simulink model "uavPackageDelivery"  (R2025b)
settings: Solver=VariableStepAuto  StartTime=0.0  StopTime=simTime  FixedStep=.005  RelTol=1e-3  EnableMultiTasking=on
undefined symbols (not defined in the file): baseMission, Newton, oaMission, Raphson, uavIC_latLon, UAVSampleTime
libraries: robotcorelib x1, uavalgslib x1, visionsinks x1, robotalgslib x1
settings Model: DataDictionary=uavPackageDeliveryDataDict.sldd  ModifiedByFormat=The MathWorks, Inc.  PauseTimes=77  Creator=The MathWorks, Inc.  LastModifiedBy=The MathWorks, Inc.
settings SolverCC: AlgebraicLoopSolver=TrustRegion  AutoInsertRateTranBlk=on  MaxZcPerStep=1.0
settings DataIOCC: LimitDataPoints=on  ReturnWorkspaceOutputs=off
settings OptimizationCC: DefaultParameterBehavior=Inlined  DefaultUnderspecifiedDataType=single  EnhancedBackFolding=on  PassReuseOutputArgsThreshold=0.0  MaxStackSize=64  OptimizeBlockOrder=speed  DifferentSizesBufferReuse=on  OptimizationCustomize=off
settings DebuggingCC: ParameterPrecisionLossMsg=none  ParameterTunabilityLossMsg=error  UnconnectedInputMsg=warning  UnconnectedOutputMsg=warning  UnconnectedLineMsg=warning  AllowSymbolicDim=off  SFUnexpectedBacktrackingDiag=warning  SFNoUnconditionalDefaultTransitionDiag=warning  SFExecutionAtInitializationDiag=none  ArithmeticOperatorsInVariantConditions=warning
settings HardwareCC: ProdBitPerPointer=32.0  ProdBitPerSizeT=32.0  ProdBitPerPtrDiffT=32.0  ProdLargestAtomicFloat=None  ProdIntDivRoundTo=Undefined  ProdEndianess=Unspecified  ProdWordSize=32.0  ProdHWDeviceType=Generic->Unspecified (assume 32-bit Generic)
settings ModelReferenceCC: EnableRefExpFcnMdlSchedulingChecks=on  PropagateSignalLabelsOutOfModel=off
settings SFSimCC: SimUseLocalCustomCode=off  SimParseCustomCode=off  CustomCodeUndefinedFunction=UseInterfaceOnly
settings RTWCC: GenerateReport=on  RTWUseLocalCustomCode=off  LaunchReport=on  GPUComputeCapability=3.5  DLArmComputeVersion=19.05
settings CodeAppCC: ForceParamTrailComments=on  OperatorAnnotations=on
settings GRTTargetCC: TargetLangStandard=C89/C90 (ANSI)
settings ConfigComp: CovMetricSettings=dw  CovSaveCumulativeToWorkspaceVar=on  CovSaveSingleToWorkspaceVar=on  CovExternalEMLEnable=off

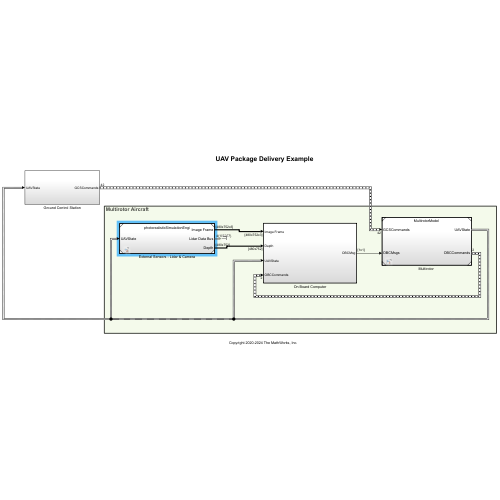
[thumbnail: Simulink's stored preview of the top-level diagram]
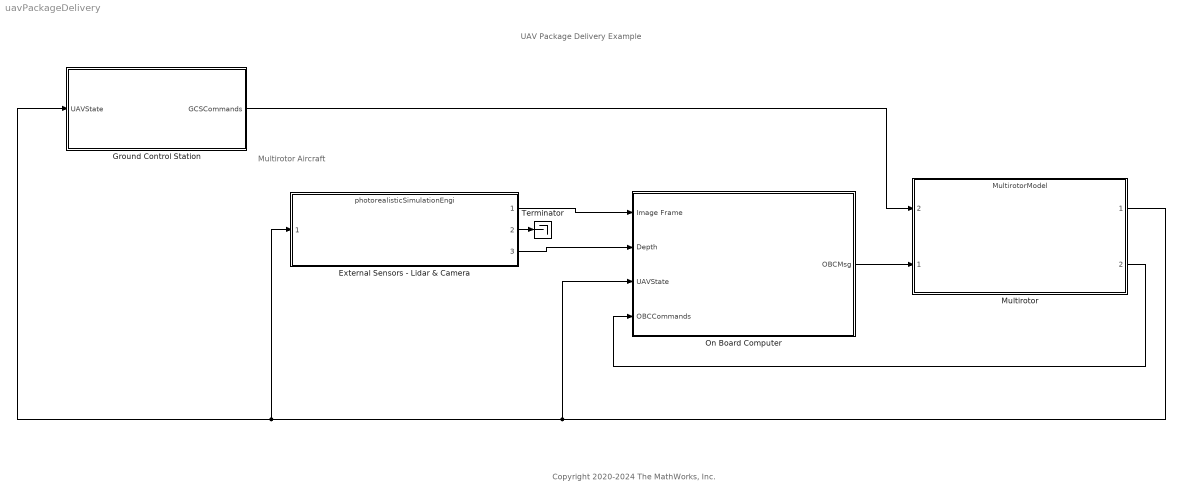
== system uavPackageDelivery ==
  note: Multirotor Aircraft
  note: UAV Package Delivery Example
  note: Copyright 2020-2024 The MathWorks, Inc.
  External Sensors - Lidar & Camera : ModelReference  ModelNameDialog=photorealisticSimulationEngi.slx  SimulationMode=Normal  ModelReferenceVersion=11.7
  Ground Control Station : Subsystem
  "Multirotor " : ModelReference  ModelNameDialog=MultirotorModel  SimulationMode=Normal  ModelReferenceVersion=12.1
      settings: PortSchema="{\"entries\":[{\"content\":{\"sides\":[{\"content\":{\"connectorIds\":[\"In2\",\"In1\"]},\"type\":\"ConnectorPlacement.EquallySpacedRectSide\",\"uuid\":\"abf53b88-b4c0-4cc3-bb4c-819ba68ade90\"},{\"content\":{\"connectorIds\":[\"Out1\",\"Out2\"],\"side\":\"RIGHT\"},\"type\":\"ConnectorPlacement.EquallySpacedRectSide\",\"uuid\":\"f1944fd3-3680-4558-bd6a-ffb0187ae725\"},{\"content\":{\"connectorIds\":[],\"side\":\"TOP\"},\"type\":\"ConnectorPlacement.EquallySpacedRectSide\",\"uuid\":\"7f686bac-a1b4-4e90-bc1f-e4dd6e8ae5c6\"}]},\"type\":\"ConnectorPlacement.EquallySpacedConnector\",\"uuid\":\"3f45c06a-90ee-44cf-add7-da13163a6845\"}],\"packageUris\":[\"http://schema.mathworks.com/mf0/Connector/19700101\"],\"version\":\"1.0\"}"
  On Board Computer : Subsystem  TreatAsAtomicUnit=on
  Terminator : Terminator
  wires:
  External Sensors - Lidar & Camera/1 -> On Board Computer/1(Image Frame)
  On Board Computer/1(OBCMsg) -> "Multirotor "/1
  "Multirotor "/1 -> Ground Control Station/1(UAVState), External Sensors - Lidar & Camera/1, On Board Computer/3(UAVState)
  "Multirotor "/2 -> On Board Computer/4(OBCCommands)
  Ground Control Station/1(GCSCommands) -> "Multirotor "/2
  External Sensors - Lidar & Camera/3 -> On Board Computer/2(Depth)
  External Sensors - Lidar & Camera/2 -> Terminator/1

== system uavPackageDelivery/Ground Control Station ==
  UAVState : Inport  OutDataTypeStr=Bus: uavStateBus
  Get Flight Mission : Subsystem  Variant=on
  Rate Transition : RateTransition  OutPortSampleTime=UAVSampleTime*4
  GCSCommands : Outport
  wires:
  UAVState/1 -> Rate Transition/1
  Get Flight Mission/1("Mission ") -> GCSCommands/1
  Rate Transition/1 -> Get Flight Mission/1(UAVState)

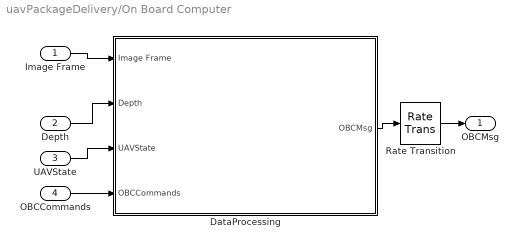
== system uavPackageDelivery/On Board Computer ==
  Image Frame : Inport
  Depth : Inport  Port=2
  UAVState : Inport  Port=3  OutDataTypeStr=Bus: uavStateBus  SampleTime=UAVSampleTime  BusOutputAsStruct=on
  OBCCommands : Inport  Port=4
  DataProcessing : Subsystem  Variant=on  PropagateVariantConditions=on
  Rate Transition : RateTransition  OutPortSampleTime=UAVSampleTime*4
  OBCMsg : Outport  OutDataTypeStr=single
  wires:
  Image Frame/1 -> DataProcessing/1(Image Frame)
  UAVState/1 -> DataProcessing/3(UAVState)
  OBCCommands/1 -> DataProcessing/4(OBCCommands)
  DataProcessing/1(OBCMsg) -> Rate Transition/1
  Rate Transition/1 -> OBCMsg/1
  Depth/1 -> DataProcessing/2(Depth)

== system uavPackageDelivery/Ground Control Station/Get Flight Mission ==
  UAVState : Inport
  QGC : Subsystem  TreatAsAtomicUnit=on  SystemSampleTime=UAVSampleTime*4  VariantControl=useQGC==1
  noQGC : Subsystem  TreatAsAtomicUnit=on  SystemSampleTime=UAVSampleTime*4  VariantControl=useQGC==0
  "Mission " : Outport

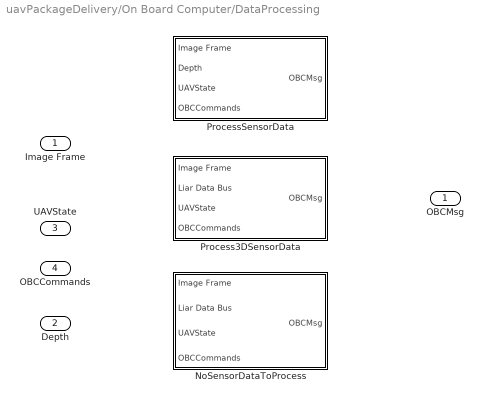
== system uavPackageDelivery/On Board Computer/DataProcessing ==
  Image Frame : Inport
  Depth : Inport  Port=2
  UAVState : Inport  Port=3  OutDataTypeStr=Bus: uavStateBus  SampleTime=0.005  BusOutputAsStruct=on
  OBCCommands : Inport  Port=4
  NoSensorDataToProcess : Subsystem  VariantControl=isPhotoRealisticSim==0
  Process3DSensorData : Subsystem  VariantControl=(isPhotoRealisticSim ==1 || isPhotoRealisticSim ==2) && guidanceType == 3
  ProcessSensorData : Subsystem  VariantControl="(isPhotoRealisticSim ==1 || isPhotoRealisticSim ==2)  && guidanceType ~= 3"
  OBCMsg : Outport  OutDataTypeStr=single  SampleTime=0.005

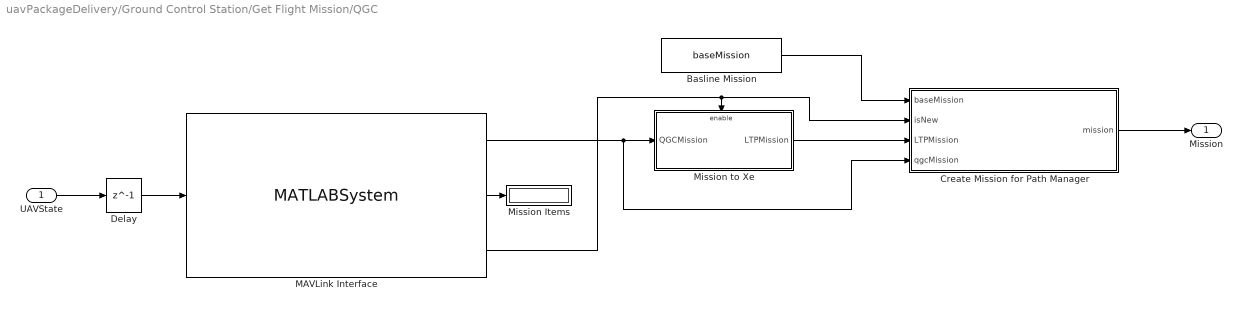
== system uavPackageDelivery/Ground Control Station/Get Flight Mission/QGC ==
  UAVState : Inport  OutDataTypeStr=Bus: uavStateBus
  Basline Mission : Constant  Value=baseMission  OutDataTypeStr=Bus: uavPathManagerBus  SampleTime=-1
  Create Mission for Path Manager : MATLAB Function  TreatAsAtomicUnit=on
  Delay : Delay  DelayLength=1
  MAVLink Interface : MATLABSystem  System=MAVLinkInterface  GCSPort=14550  MaxMissionLength=42  homeLatitude=uavIC_latLon(1)  homeLongitude=uavIC_latLon(2)
      mask Type: MAVLinkInterface
  Mission Items : Display
  Mission to Xe : Subsystem
  Mission : Outport  OutDataTypeStr=Bus: uavPathManagerBus
  wires:
  MAVLink Interface/3 -> Create Mission for Path Manager/2(isNew), Mission to Xe/Enable
  Basline Mission/1 -> Create Mission for Path Manager/1(baseMission)
  Mission to Xe/1(LTPMission) -> Create Mission for Path Manager/3(LTPMission)
  Create Mission for Path Manager/1(mission) -> Mission/1
  MAVLink Interface/1 -> Mission to Xe/1(QGCMission), Create Mission for Path Manager/4(qgcMission)
  Delay/1 -> MAVLink Interface/1
  UAVState/1 -> Delay/1
  MAVLink Interface/2 -> Mission Items/1

== system uavPackageDelivery/Ground Control Station/Get Flight Mission/noQGC ==
  Variant Source : VariantSource  VariantControls={guidanceType==1, guidanceType==2 || guidanceType == 3}
  Waypoints : Constant  Value=baseMission  OutDataTypeStr=Bus: uavPathManagerBus  SampleTime=-1
  Waypoints1 : Constant  Value=oaMission  OutDataTypeStr=Bus: uavPathManagerBus  SampleTime=-1
  Mission : Outport
  wires:
  Waypoints/1 -> Variant Source/1
  Waypoints1/1 -> Variant Source/2
  Variant Source/1 -> Mission/1

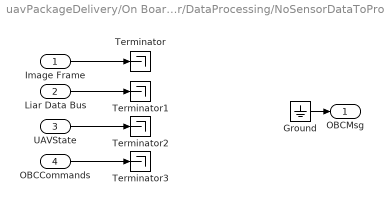
== system uavPackageDelivery/On Board Computer/DataProcessing/NoSensorDataToProcess ==
  Image Frame : Inport
  "Liar Data Bus " : Inport  Port=2
  UAVState : Inport  Port=3  OutDataTypeStr=Bus: uavStateBus  SampleTime=UAVSampleTime  BusOutputAsStruct=on
  OBCCommands : Inport  Port=4
  Ground : Ground
  Terminator{,1..3} (4 alike) : Terminator
  OBCMsg : Outport  OutDataTypeStr=single  SampleTime=UAVSampleTime
  wires:
  Ground/1 -> OBCMsg/1
  Image Frame/1 -> Terminator/1
  "Liar Data Bus "/1 -> Terminator1/1
  UAVState/1 -> Terminator2/1
  OBCCommands/1 -> Terminator3/1

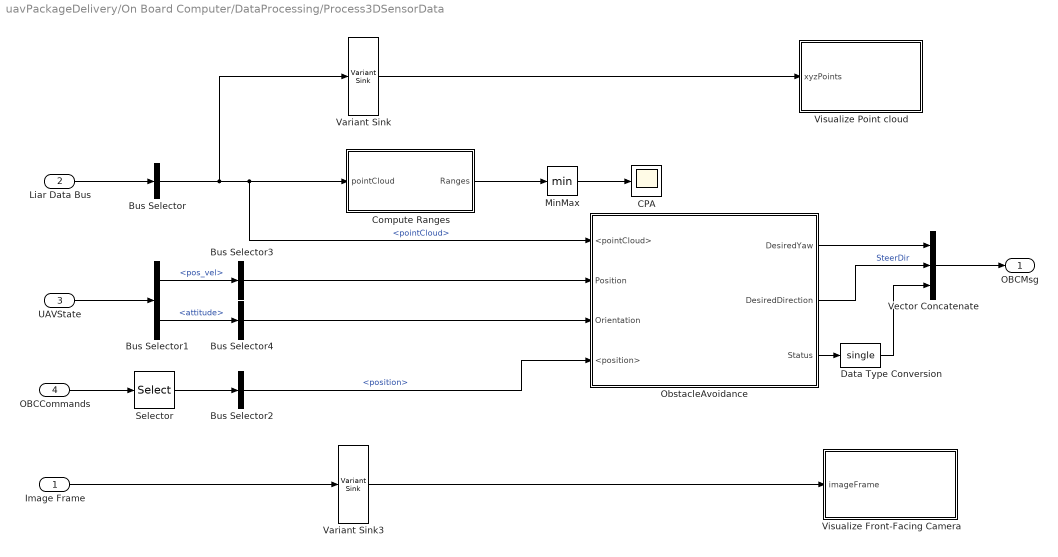
== system uavPackageDelivery/On Board Computer/DataProcessing/Process3DSensorData ==
  Image Frame : Inport
  "Liar Data Bus " : Inport  Port=2  SampleTime=0.5
  UAVState : Inport  Port=3  OutDataTypeStr=Bus: uavStateBus  SampleTime=0.5  BusOutputAsStruct=on
  OBCCommands : Inport  Port=4  SampleTime=0.5
  Bus Selector : BusSelector  OutputSignals=pointCloud
  Bus Selector1 : BusSelector  OutputSignals=pos_vel,attitude
  Bus Selector2 : BusSelector  OutputSignals=position
  Bus Selector3 : BusSelector  OutputSignals=x,y,z  OutputAsBus=on
  Bus Selector4 : BusSelector  OutputSignals=yaw,pitch,roll  OutputAsBus=on
  CPA : Scope
      settings: TimeSpan=200  ActiveDisplayYMinimum=-1.62863  ActiveDisplayYMaximum=22.80719
  Compute Ranges : Subsystem
  Data Type Conversion : DataTypeConversion  OutDataTypeStr=single  SaturateOnIntegerOverflow=off  RndMeth=Floor
  MinMax : MinMax
  ObstacleAvoidance : Subsystem
  Selector : Selector  InputPortWidth=2  IndexOptions=Index vector (dialog)  Indices=[2]  OutputSizes=1
  Variant Sink : VariantSink  VariantControls={showLidarPointCloud ==1}
      settings: AllowZeroVariantControls=on
  Variant Sink3 : VariantSink  VariantControls={showVideoViewer == 1}
      settings: AllowZeroVariantControls=on
  Vector Concatenate : Concatenate  NumInputs=3
  Visualize Front-Facing Camera : MATLAB Function  TreatAsAtomicUnit=on
  Visualize Point cloud : MATLAB Function  StopFcn=|  TreatAsAtomicUnit=on
      | playerFigure = findall(groot,'type','figure','name','Point Cloud Player');
      | 
      | if ~isempty(playerFigure)
      |     playerFigure = playerFigure(end);
      |     if isvalid(playerFigure)
      |         close(playerFigure);
      |     end
      | end
  OBCMsg : Outport  OutDataTypeStr=single  SampleTime=0.005
  wires:
  Bus Selector/1 -> ObstacleAvoidance/1(<pointCloud>), Compute Ranges/1(pointCloud), Variant Sink/1  "<pointCloud>"
  Bus Selector1/2 -> Bus Selector4/1  "<attitude>"
  Variant Sink/1 -> Visualize Point cloud/1(xyzPoints)
  Selector/1 -> Bus Selector2/1
  MinMax/1 -> CPA/1
  Image Frame/1 -> Variant Sink3/1
  Bus Selector1/1 -> Bus Selector3/1  "<pos_vel>"
  UAVState/1 -> Bus Selector1/1
  "Liar Data Bus "/1 -> Bus Selector/1
  Vector Concatenate/1 -> OBCMsg/1
  ObstacleAvoidance/1(DesiredYaw) -> Vector Concatenate/1
  Compute Ranges/1(Ranges) -> MinMax/1
  Bus Selector4/1 -> ObstacleAvoidance/3(Orientation)
  Bus Selector3/1 -> ObstacleAvoidance/2(Position)
  Bus Selector2/1 -> ObstacleAvoidance/4(<position>)  "<position>"
  ObstacleAvoidance/2(DesiredDirection) -> Vector Concatenate/2  "SteerDir"
  OBCCommands/1 -> Selector/1
  Variant Sink3/1 -> Visualize Front-Facing Camera/1(imageFrame)
  ObstacleAvoidance/3(Status) -> Data Type Conversion/1
  Data Type Conversion/1 -> Vector Concatenate/3

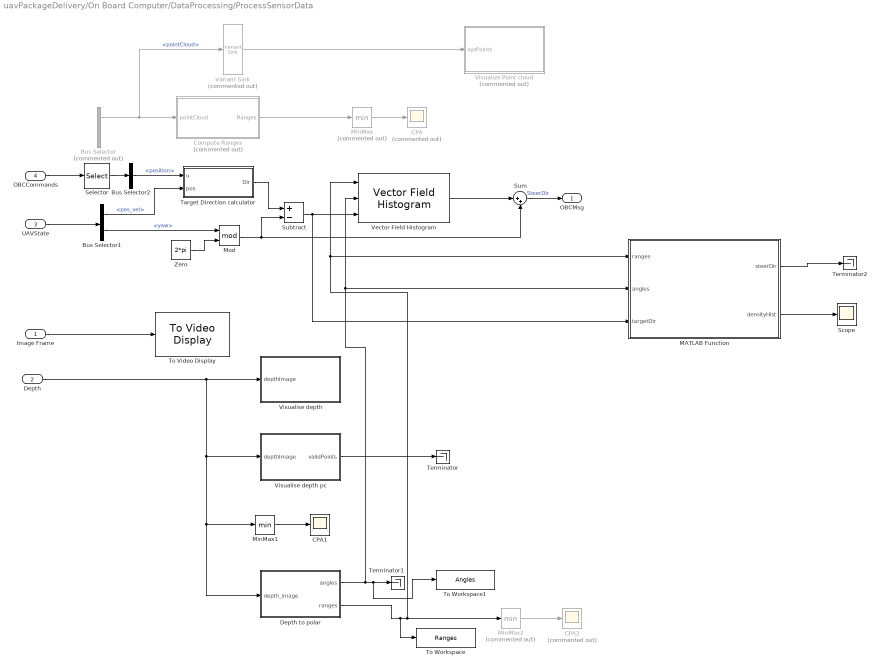
== system uavPackageDelivery/On Board Computer/DataProcessing/ProcessSensorData ==
  Image Frame : Inport
  Depth : Inport  Port=2
  UAVState : Inport  Port=3  OutDataTypeStr=Bus: uavStateBus  SampleTime=UAVSampleTime*10  BusOutputAsStruct=on
  OBCCommands : Inport  Port=4  SampleTime=UAVSampleTime*10
  Bus Selector : BusSelector  Commented=on  OutputSignals=pointCloud,lidarAngles
  Bus Selector1 : BusSelector  OutputSignals=pos_vel,attitude.yaw
  Bus Selector2 : BusSelector  OutputSignals=position
  CPA : Scope  Commented=on
      settings: TimeSpan=200  ActiveDisplayYMinimum=3.83822  ActiveDisplayYMaximum=27.99117
  CPA1 : Scope
      settings: TimeSpan=200  ActiveDisplayYMinimum=-196.83407666584111  ActiveDisplayYMaximum=881.58454530198583  DataLoggingVariableName=ScopeData2
  CPA2 : Scope  Commented=on
      settings: TimeSpan=200  ActiveDisplayYMinimum=3.2265628490796132  ActiveDisplayYMaximum=57.375866008315271  DataLoggingVariableName=ScopeData3
  Compute Ranges : Subsystem  Commented=on
  "Depth to polar " : MATLAB Function  StopFcn=|  TreatAsAtomicUnit=on
      | playerFigure = findall(groot,'type','figure','name','Point Cloud Player');
      | 
      | if ~isempty(playerFigure)
      |     playerFigure = playerFigure(end);
      |     if isvalid(playerFigure)
      |         close(playerFigure);
      |     end
      | end
  MATLAB Function : MATLAB Function  TreatAsAtomicUnit=on
  MinMax : MinMax  Commented=on
  MinMax1 : MinMax
  MinMax2 : MinMax  Commented=on  ZeroCross=off
  Mod : Math  Operator=mod
  Scope : Scope
      settings: ActiveDisplayYMinimum=-38.316782935620068  ActiveDisplayYMaximum=95.601752317315714  DataLoggingVariableName=ScopeData6
  Selector : Selector  InputPortWidth=2  IndexOptions=Index vector (dialog)  Indices=[2]  OutputSizes=1
  Subtract : Sum  Inputs=+-
  Sum : Sum  Inputs=|++  AccumDataTypeStr=single
  Target Direction calculator : MATLAB Function  TreatAsAtomicUnit=on
  Terminator : Terminator
  Terminator1 : Terminator
  Terminator2 : Terminator
  To Video Display : visionsinks/To Video Display  windowSizeMode=Normal  openAtMdlStart=on  fullScreen=off  videoWindowX=616  videoWindowY=477  saveWindowSize=off  videoWindowWidth=752  videoWindowHeight=480  inputColorFormat=RGB  inputType=Obsolete  imagePorts=One multidimensional signal  OutputDevice=On-screen video monitor  dataOrg=Column-major  isWindowOpen=off
  To Workspace : ToWorkspace  VariableName=Ranges  SaveFormat=Timeseries  SampleTime=-1
  To Workspace1 : ToWorkspace  VariableName=Angles  SaveFormat=Timeseries  SampleTime=-1
  Variant Sink : VariantSink  Commented=on  VariantControls={showLidarPointCloud ==1}
      settings: AllowZeroVariantControls=on
  Vector Field Histogram : robotalgslib/Vector Field Histogram  NumAngularSectors=360  DistanceLimits=[ 0.5 ,10 ]  HistogramThresholds=[ 5, 10 ]  RobotRadius=.5  SafetyDistance=5  MinTurningRadius=2  SimulateUsing=Code generation  TargetDirectionWeight=5  CurrentDirectionWeight=2  PreviousDirectionWeight=2
  "Visualise depth " : MATLAB Function  StopFcn=|  TreatAsAtomicUnit=on
      | playerFigure = findall(groot,'type','figure','name','Point Cloud Player');
      | 
      | if ~isempty(playerFigure)
      |     playerFigure = playerFigure(end);
      |     if isvalid(playerFigure)
      |         close(playerFigure);
      |     end
      | end
  Visualise depth pc : MATLAB Function  StopFcn=|  TreatAsAtomicUnit=on
      | playerFigure = findall(groot,'type','figure','name','Point Cloud Player');
      | 
      | if ~isempty(playerFigure)
      |     playerFigure = playerFigure(end);
      |     if isvalid(playerFigure)
      |         close(playerFigure);
      |     end
      | end
  Visualize Point cloud : MATLAB Function  Commented=on  StopFcn=|  TreatAsAtomicUnit=on
      | playerFigure = findall(groot,'type','figure','name','Point Cloud Player');
      | 
      | if ~isempty(playerFigure)
      |     playerFigure = playerFigure(end);
      |     if isvalid(playerFigure)
      |         close(playerFigure);
      |     end
      | end
  Zero : Constant  Value=2*pi  OutDataTypeStr=Inherit: Inherit via back propagation
  OBCMsg : Outport  OutDataTypeStr=single  SampleTime=0.005
  wires:
  UAVState/1 -> Bus Selector1/1
  Subtract/1 -> MATLAB Function/3(targetDir), Vector Field Histogram/3
  Target Direction calculator/1(Dir) -> Subtract/1
  Bus Selector1/2 -> Mod/1  "<yaw>"
  Bus Selector2/1 -> Target Direction calculator/1(u)  "<position>"
  Image Frame/1 -> To Video Display/1
  Zero/1 -> Mod/2
  Selector/1 -> Bus Selector2/1
  Compute Ranges/1(Ranges) -> MinMax/1
  Bus Selector/1 -> Compute Ranges/1(pointCloud), Variant Sink/1  "<pointCloud>"
  OBCCommands/1 -> Selector/1
  MinMax/1 -> CPA/1
  Sum/1 -> OBCMsg/1  "SteerDir"
  Bus Selector1/1 -> Target Direction calculator/2(pos)  "<pos_vel>"
  Variant Sink/1 -> Visualize Point cloud/1(xyzPoints)
  Mod/1 -> Sum/2, Subtract/2
  Vector Field Histogram/1 -> Sum/1
  Depth/1 -> "Depth to polar "/1(depth_image), MinMax1/1, Visualise depth pc/1(depthImage), "Visualise depth "/1(depthImage)
  MinMax1/1 -> CPA1/1
  Visualise depth pc/1(validPoints) -> Terminator/1
  MinMax2/1 -> CPA2/1
  "Depth to polar "/1(angles) -> Vector Field Histogram/2, MATLAB Function/2(angles), To Workspace1/1, Terminator1/1
  "Depth to polar "/2(ranges) -> To Workspace/1, MinMax2/1, Vector Field Histogram/1, MATLAB Function/1(ranges)
  MATLAB Function/2(densityHist) -> Scope/1
  MATLAB Function/1(steerDir) -> Terminator2/1

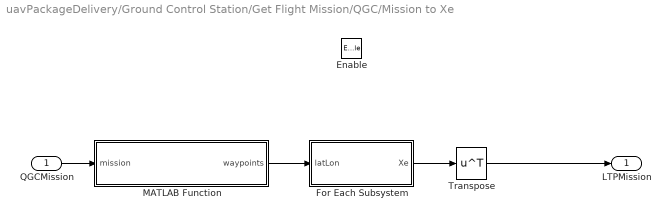
== system uavPackageDelivery/Ground Control Station/Get Flight Mission/QGC/Mission to Xe ==
  QGCMission : Inport
  Enable : EnablePort
  For Each Subsystem : Subsystem  TreatAsAtomicUnit=on
  MATLAB Function : MATLAB Function  TreatAsAtomicUnit=on
  Transpose : Math  Operator=transpose
  LTPMission : Outport
  wires:
  For Each Subsystem/1(Xe) -> Transpose/1
  MATLAB Function/1(waypoints) -> For Each Subsystem/1(latLon)
  QGCMission/1 -> MATLAB Function/1(mission)
  Transpose/1 -> LTPMission/1

== system uavPackageDelivery/On Board Computer/DataProcessing/Process3DSensorData/Compute Ranges ==
  pointCloud : Inport
  For Each Subsystem1 : Subsystem  TreatAsAtomicUnit=on
  Reshape1 : Reshape  OutputDimensions=1083
  Ranges : Outport
  wires:
  For Each Subsystem1/1(Out1) -> Reshape1/1
  pointCloud/1 -> For Each Subsystem1/1(In1)
  Reshape1/1 -> Ranges/1

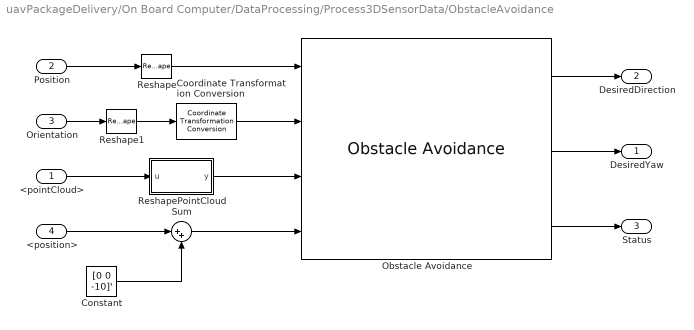
== system uavPackageDelivery/On Board Computer/DataProcessing/Process3DSensorData/ObstacleAvoidance ==
  <pointCloud> : Inport
  Position : Inport  Port=2
  Orientation : Inport  Port=3
  <position> : Inport  Port=4
  Constant : Constant  Value=[0 0 -10]'  VectorParams1D=off  OutDataTypeStr=single
  Coordinate Transformation Conversion : robotcorelib/Coordinate Transformation Conversion  InputRepresentation=Euler Angles  InputEulerSequence=ZYX  ShowTrVecInputPort=on  OutputRepresentation=Quaternion  OutputEulerSequence=ZYX  ShowTrVecOutputPort=on  SimulateUsing=Code generation
  Obstacle Avoidance : uavalgslib/Obstacle Avoidance  DistanceLimits=[ 0.2, 30 ]  HorizontalSensorFOV=[ -180, 180 ]  VerticalSensorFOV=[ -20, 20 ]  SensorLocation=[ 0, 0, -0.4 ]  SensorOrientation=[ 180, 0, 0 ]  VehicleRadius=0.5  SafetyDistance=0.75  SimulateUsing=Code generation  HistRes=5  WindowSize=1  HistogramThreshold=1  MaxAge=5  TargetDirectionWeight=3  CurrentDirectionWeight=1  PreviousDirectionWeight=2
  Reshape : Reshape  OutputDimensionality=Column vector (2-D)
  Reshape1 : Reshape  OutputDimensionality=Column vector (2-D)
  ReshapePointCloud : MATLAB Function  TreatAsAtomicUnit=on
  Sum : Sum  Inputs=|++
  DesiredYaw : Outport
  DesiredDirection : Outport  Port=2
  Status : Outport  Port=3
  wires:
  Obstacle Avoidance/1 -> DesiredDirection/1
  Obstacle Avoidance/3 -> Status/1
  <pointCloud>/1 -> ReshapePointCloud/1(u)
  Obstacle Avoidance/2 -> DesiredYaw/1
  Position/1 -> Reshape/1
  <position>/1 -> Sum/1
  Orientation/1 -> Reshape1/1
  Reshape/1 -> Obstacle Avoidance/1
  Reshape1/1 -> Coordinate Transformation Conversion/1
  ReshapePointCloud/1(y) -> Obstacle Avoidance/3
  Sum/1 -> Obstacle Avoidance/4
  Constant/1 -> Sum/2
  Coordinate Transformation Conversion/1 -> Obstacle Avoidance/2

== system uavPackageDelivery/On Board Computer/DataProcessing/ProcessSensorData/Compute Ranges ==
  pointCloud : Inport
  For Each Subsystem : Subsystem  TreatAsAtomicUnit=on
  Reshape : Reshape  OutputDimensionality=Customize  OutputDimensions=[1083 3]
  Reshape1 : Reshape  OutputDimensions=1083
  Selector1 : Selector  NumberOfDimensions=3  InputPortWidth=3  IndexOptions=Index vector (dialog),Select all,Select all  Indices=16,1,1  OutputSizes=1,1,1
  Ranges : Outport
  wires:
  For Each Subsystem/1(Out1) -> Reshape1/1
  Selector1/1 -> Reshape/1
  pointCloud/1 -> Selector1/1
  Reshape/1 -> For Each Subsystem/1(In1)
  Reshape1/1 -> Ranges/1

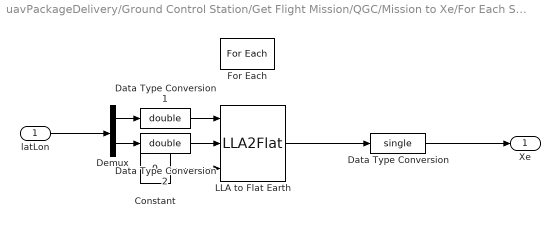
== system uavPackageDelivery/Ground Control Station/Get Flight Mission/QGC/Mission to Xe/For Each Subsystem ==
  latLon : Inport  Partition=on  PartitionDimension=1  PartitionWidth=1  PartitionOffset=0
  Constant : Constant  Value=0  OutDataTypeStr=double
  Data Type Conversion : DataTypeConversion  OutDataTypeStr=single  SaturateOnIntegerOverflow=off  RndMeth=Floor
  Data Type Conversion1 : DataTypeConversion  OutDataTypeStr=double  SaturateOnIntegerOverflow=off  RndMeth=Floor
  Data Type Conversion2 : DataTypeConversion  OutDataTypeStr=double  SaturateOnIntegerOverflow=off  RndMeth=Floor
  Demux : Demux  Outputs=[2 1]
  For Each : ForEach  DisableCoverage=on
  LLA to Flat Earth : LLA2Flat  R=6378137  LL0=uavIC_latLon
  Xe : Outport  ConcatenationDimension=2
  wires:
  LLA to Flat Earth/1 -> Data Type Conversion/1
  Demux/2 -> Data Type Conversion2/1
  Demux/1 -> Data Type Conversion1/1
  latLon/1 -> Demux/1
  Constant/1 -> LLA to Flat Earth/3
  Data Type Conversion/1 -> Xe/1
  Data Type Conversion1/1 -> LLA to Flat Earth/1
  Data Type Conversion2/1 -> LLA to Flat Earth/2

== system uavPackageDelivery/On Board Computer/DataProcessing/Process3DSensorData/Compute Ranges/For Each Subsystem1 ==
  In1 : Inport  Partition=on  PartitionDimension=1  PartitionWidth=1  PartitionOffset=0
  For Each Horizontal Slice : ForEach  DisableCoverage=on
  Process each Horizontal Slice : Subsystem  TreatAsAtomicUnit=on
  Reshape : Reshape
  Out1 : Outport  ConcatenationDimension=1
  wires:
  In1/1 -> Process each Horizontal Slice/1(pointCloud)
  Process each Horizontal Slice/1(Out1) -> Reshape/1
  Reshape/1 -> Out1/1

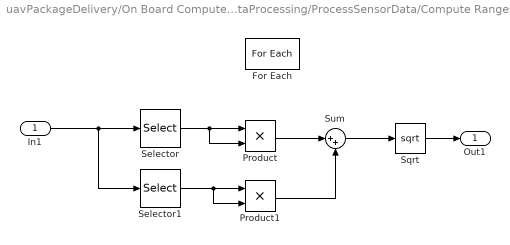
== system uavPackageDelivery/On Board Computer/DataProcessing/ProcessSensorData/Compute Ranges/For Each Subsystem ==
  In1 : Inport  Partition=on  PartitionDimension=1  PartitionWidth=1  PartitionOffset=0
  For Each : ForEach  DisableCoverage=on
  Product : Product
  Product1 : Product
  Selector : Selector  InputPortWidth=3  IndexOptions=Index vector (dialog)  Indices=[1]  OutputSizes=1
  Selector1 : Selector  InputPortWidth=3  IndexOptions=Index vector (dialog)  Indices=[2]  OutputSizes=1
  Sqrt : Sqrt  OutputSignalType=real  OutDataTypeStr=single  IntermediateResultsDataTypeStr=single  AlgorithmType=Newton-Raphson
  Sum : Sum  Inputs=|++
  Out1 : Outport  ConcatenationDimension=1
  wires:
  In1/1 -> Selector1/1, Selector/1
  Selector/1 -> Product/2, Product/1
  Selector1/1 -> Product1/2, Product1/1
  Product/1 -> Sum/1
  Product1/1 -> Sum/2
  Sum/1 -> Sqrt/1
  Sqrt/1 -> Out1/1

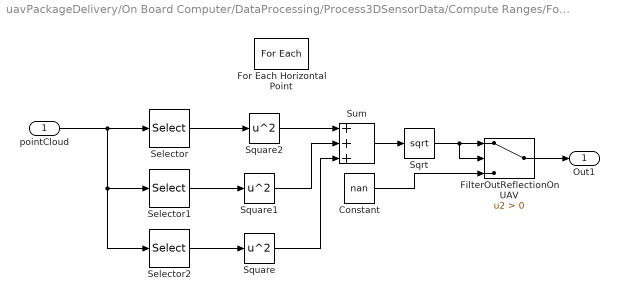
== system uavPackageDelivery/On Board Computer/DataProcessing/Process3DSensorData/Compute Ranges/For Each Subsystem1/Process each Horizontal Slice ==
  pointCloud : Inport  Partition=on  PartitionDimension=2  PartitionWidth=1  PartitionOffset=0
  Constant : Constant  Value=nan
  FilterOutReflectionOnUAV : Switch  Criteria=u2 > Threshold  SaturateOnIntegerOverflow=off  InputSameDT=off
  For Each Horizontal Point : ForEach  DisableCoverage=on
  Selector : Selector  NumberOfDimensions=3  InputPortWidth=3  IndexOptions=Index vector (dialog),Index vector (dialog),Index vector (dialog)  Indices=1,1,1  OutputSizes=1,1,1
  Selector1 : Selector  NumberOfDimensions=3  InputPortWidth=3  IndexOptions=Index vector (dialog),Index vector (dialog),Index vector (dialog)  Indices=1,1,2  OutputSizes=1,1,1
  Selector2 : Selector  NumberOfDimensions=3  InputPortWidth=3  IndexOptions=Index vector (dialog),Index vector (dialog),Index vector (dialog)  Indices=1,1,3  OutputSizes=1,1,1
  Sqrt : Sqrt  OutputSignalType=real  OutDataTypeStr=single  IntermediateResultsDataTypeStr=single  AlgorithmType=Newton-Raphson
  Square : Math  Operator=square
  Square1 : Math  Operator=square
  Square2 : Math  Operator=square
  Sum : Sum  Inputs=+++
  Out1 : Outport  ConcatenationDimension=1
  wires:
  pointCloud/1 -> Selector2/1, Selector1/1, Selector/1
  Selector/1 -> Square2/1
  Selector1/1 -> Square1/1
  Square2/1 -> Sum/1
  Square1/1 -> Sum/2
  Sum/1 -> Sqrt/1
  Sqrt/1 -> FilterOutReflectionOnUAV/1, FilterOutReflectionOnUAV/2
  Selector2/1 -> Square/1
  Square/1 -> Sum/3
  FilterOutReflectionOnUAV/1 -> Out1/1
  Constant/1 -> FilterOutReflectionOnUAV/3

== matlab function uavPackageDelivery/On Board Computer/DataProcessing/ProcessSensorData/Visualise depth  ==
  data: depthImage input
function visualizeDepthImage(depthImage)
% VISUALIZEDEPTHIMAGE  Display a depth map with automatic scaling.
%
% Usage:
%   visualizeDepthImage(depthImage)
%
% Example:
%   depth = imread('depth_image.png');
%   visualizeDepthImage(depth);

    coder.extrinsic('figure', 'axes', 'imagesc', 'colormap', 'colorbar', 'ylabel', 'title', 'drawnow', 'isvalid');
    
    persistent figHandle axHandle cbHandle;
    
    % Convert to double precision
    depthImage = double(depthImage);
    
    % Replace invalid or missing values with NaN
    depthImage(depthImage == 0) = NaN;
    
    % Determine display limits automatically
    maxDepth = min(150, max(depthImage(:), [], 'omitnan'));  % cap far values
    depthImage(depthImage > maxDepth) = maxDepth;
    
    % Create figure and axes on first call - use only isempty for validation
    if isempty(figHandle)
        figHandle = figure('Name', 'Depth Image (Jet)', 'NumberTitle', 'off');
        axHandle = axes('Parent', figHandle);
        axis(axHandle, 'image', 'off');
        colormap(axHandle, 'jet');
        cbHandle = colorbar(axHandle);
        ylabel(cbHandle, 'Depth (metres)');
    else
        % For subsequent calls, check if figure still exists using isempty only
        % If figure was closed, the handle becomes invalid but we can only check isempty
        % In practice, the figure will persist until explicitly closed
        if isempty(figHandle)
            % Recreate if needed (though this case should be rare)
            figHandle = figure('Name', 'Depth Image (Jet)', 'NumberTitle', 'off');
            axHandle = axes('Parent', figHandle);
            axis(axHandle, 'image', 'off');
            colormap(axHandle, 'jet');
            cbHandle = colorbar(axHandle);
            ylabel(cbHandle, 'Depth (metres)');
        end
    end
    
    % Update the image
    imagesc(axHandle, depthImage, [0 maxDepth]);
    title(axHandle, sprintf('Depth Image (Clipped at %.1f m)', maxDepth));
    
    % Ensure colorbar exists
    if isempty(cbHandle)
        cbHandle = colorbar(axHandle);
        ylabel(cbHandle, 'Depth (metres)');
    end
    
    drawnow;
end

== matlab function uavPackageDelivery/On Board Computer/DataProcessing/ProcessSensorData/Visualise depth pc ==
  data: depthImage input; validPoints output double size=[360960 3]
function validPoints = visualizeDepthPC(depthImage)
% VISUALIZEDEPTHPC pcfromdepth-style for 150m depth range
% Input: depthImage [480x752] with depths up to 150m
% Output: validPoints [N×3] 3D point cloud matrix

    coder.extrinsic('pointCloud', 'isOpen', 'pcplayer', 'view');
    
    persistent player;
    
    % Camera intrinsic parameters
    fx = 1109;
    fy = 1109;
    cx = 640;
    cy = 360;
    
    [height, width] = size(depthImage);
    
    % Pre-allocate point array
    maxPoints = height * width;
    points = zeros(maxPoints, 3);
    validCount = 0;
    
    % Back-project each pixel to 3D with 150m range
    for v = 1:height      % row index (y)
        for u = 1:width   % column index (x)
            Z_val = double(depthImage(v, u));
            
            % Validate depth value (0 to 150 meters)
            if Z_val > 0 && Z_val <= 150.0
                validCount = validCount + 1;
                
                % Back-project using pinhole camera model
                points(validCount, 1) = (u - cx) * Z_val / fx;  % X
                points(validCount, 2) = (v - cy) * Z_val / fy;  % Y
                points(validCount, 3) = Z_val;                  % Z
            end
        end
    end
    
    % Extract valid points only
    if validCount > 0
        validPoints = points(1:validCount, :);
    else
        validPoints = zeros(0, 3);
    end
    
    % Create pointCloud object
    ptCloud = pointCloud(validPoints);
    
    % Initialize and update pcplayer with expanded limits for 150m range
    if isempty(player)
        % Expanded limits to accommodate 150m depth
        % X and Y limits calculated based on maximum field of view
        maxX = (width - cx) * 150 / fx;   % Maximum X at 150m
        maxY = (height - cy) * 150 / fy;  % Maximum Y at 150m
        
        xlimits = [-maxX, maxX];
        ylimits = [-maxY, maxY];
        zlimits = [0, 160];  % Slightly beyond 150m for visibility
        
        player = pcplayer(xlimits, ylimits, zlimits);
    end
    
    if ~isempty(player) && isOpen(player) && validCount > 0
        view(player, validPoints);
    end
end

== matlab function uavPackageDelivery/On Board Computer/DataProcessing/Process3DSensorData/ObstacleAvoidance/ReshapePointCloud ==
  data: u input; y output
function y = fcn(u)
y = [reshape(u(:,:,1),[],1), reshape(u(:,:,2),[],1), reshape(u(:,:,3),[],1)];

== matlab function uavPackageDelivery/On Board Computer/DataProcessing/Process3DSensorData/Visualize Front-Facing Camera ==
  data: imageFrame input
function plotImageFrame(imageFrame)

coder.extrinsic('ishandle','image');

persistent fig;

if isempty(fig)
    fig = figure();
    ax = newplot(fig);
    title(ax, 'Front-facing camera');
end

if ~isempty(fig) && ishandle(fig)
    ax = newplot(fig);
    image(ax, imageFrame);
    axis(ax, 'off');
end

== matlab function uavPackageDelivery/On Board Computer/DataProcessing/Process3DSensorData/Visualize Point cloud ==
  data: xyzPoints input
function VisualizePointCloud(xyzPoints)
%VisualizePointCloud Display point cloud

coder.extrinsic('isOpen', 'pcplayer')

persistent player;

if isempty(player)
    % Configure axes limits
    xlimits = [-90 90];
    ylimits = [-90 90];
    zlimits = [ -50 50];
    
    % Create a streaming Lidar viewer
    player = pcplayer(xlimits, ylimits, zlimits);
end

if ~isempty(player) && isOpen(player)
    view(player, xyzPoints);
end

== matlab function uavPackageDelivery/Ground Control Station/Get Flight Mission/QGC/Mission to Xe/MATLAB Function ==
  data: mission input Bus: uavPathManagerBus size=42; waypoints output single size=[42 3]
function waypoints  = buildUAVMission(mission)
%
waypoints = single(zeros(42,3));

for i=1:length(mission)
    waypoints(i,1:3) = mission(i).position;
end

end

== matlab function uavPackageDelivery/Ground Control Station/Get Flight Mission/QGC/Create Mission for Path Manager ==
  data: baseMission input Bus: uavPathManagerBus size=42; isNew input size=1; LTPMission input size=[42 3]; mission output Bus: uavPathManagerBus size=42; qgcMission input Bus: uavPathManagerBus size=42
function mission = generateWaypointStream(baseMission, isNew, LTPMission, qgcMission)
persistent UAVMission

%% If we got a new mission
if (isNew == true)
    UAVMission = baseMission; % Initialize structure
    for ii=1:42
        if LTPMission(ii,2) < 7275326
            UAVMission(ii).position = LTPMission(ii,:)';
            y = isnan(qgcMission(ii).params);
            UAVMission(ii).params = qgcMission(ii).params;
            if sum(y)>0
                UAVMission(ii).params(y) = single(0);
            end
            UAVMission(ii).mode = mavlinkToPlannerType(qgcMission(ii).mode);
        end
    end
end

% If no mission received yet, create a loiter/hold mission
if isempty(UAVMission)
    UAVMission = baseMission; % Use baseMission as template to get correct size
    for ii=1:42
        UAVMission(ii).position =single([0; 0; 0]); % Or use current UAV position
        UAVMission(ii).params = single([0; 0; 0; 0]); % Default params
        UAVMission(ii).mode = uint8(3); % Loiter mode
    end
end


mission = UAVMission;

end

function plannerType = mavlinkToPlannerType(mavlinkType)
% see enum name="MAV_CMD" in common.xml for values.
switch mavlinkType
    case 16 %MAV_CMD_NAV_WAYPOINT
        plannerType = uint8(2);
    case 18 %MAV_CMD_NAV_LOITER_TURNS
        plannerType = uint8(3);
    case 21 %MAV_CMD_NAV_LAND
        plannerType = uint8(4);
    case 22 %MAV_CMD_NAV_TAKEOFF
        plannerType = uint8(1);
    otherwise %this will likely error out to signal something unexpected
        plannerType = uint8(0);
end
end

== matlab function uavPackageDelivery/On Board Computer/DataProcessing/ProcessSensorData/Target Direction calculator ==
  data: u input; Dir output; pos input
function Dir = TargetDir(u, pos)

Dir = atan2(u(2)-pos.y, u(1)-pos.x);

end

== matlab function uavPackageDelivery/On Board Computer/DataProcessing/ProcessSensorData/Depth to polar  ==
  data: depth_image input; angles output size=[1275 1]; ranges output size=[1275]
function [angles, ranges] = depth_to_polar(depth_image)
% Convert depth image to polar coordinates (angles and ranges) for VFH
%
% Inputs:
%   depth_image: 480x752 matrix of depth values in meters
%
% Outputs:
%   angles: Nx1 single vector of horizontal angles (radians)
%   ranges: Nx1 single vector of ranges (meters)
    %% Camera Parameters
    fx = single(1109);              % Focal length x (pixels)
    fy = single(1109);              % Focal length y (pixels)
    cx = single(640);               % Optical center x (pixels)
    cy = single(360);               % Optical center y (pixels)
    img_height = 480;
    img_width = 752;
    
    % Camera translation from robot center [forward, left, up] (m)
    cam_translation = single([0.15, 0, -0.15]);
    
    %% Distance limits
    d_min = single(0.15);           % Minimum valid distance (m)
    d_max = single(150);            % Maximum valid distance (m)
    
    %% Vertical cropping parameters
    v_start = 120;  % Start from row 120
    v_end = 360;    % End at row 360
    
    %% Downsample for performance
    step_u = 15;  % Process every 15th pixel horizontally
    step_v = 10;  % Process every 10th pixel vertically
    
    %% Calculate exact output size
    num_v = floor((v_end - v_start) / step_v) + 1;
    num_u = floor((img_width - 1) / step_u) + 1;
    max_points = num_v * num_u;  % Should be 1275
    
    %% Preallocate arrays (single precision)
    angles = single(zeros(max_points, 1));
    ranges = single(zeros(max_points, 1));
    count = 0;
    
    %% Process each pixel in depth image
    for v = v_start:step_v:v_end
        for u = 1:step_u:img_width
            depth = single(depth_image(v, u));
            
            % Skip invalid depths
            if isnan(depth) || isinf(depth) || depth < d_min || depth > d_max
                continue;
            end
            
            % Convert pixel to normalized camera coordinates
            x_norm = (u - cx) / fx;
            y_norm = (v - cy) / fy;
            
            % Convert to 3D point in camera frame
            x_cam = x_norm * depth;
            y_cam = y_norm * depth;
            z_cam = depth;
            
            % Transform to robot frame
            x_robot = z_cam + cam_translation(1);   % forward
            y_robot = -x_cam + cam_translation(2);  % left
            z_robot = -y_cam + cam_translation(3);  % up
            
            % Calculate angle and range
            angle_rad = atan2(y_robot, x_robot);
            range_m = sqrt(x_robot^2 + y_robot^2);
            
            % Store valid measurements
            if range_m >= d_min && range_m <= d_max
                count = count + 1;
                angles(count) = angle_rad;
                ranges(count) = range_m;
            end
        end
    end
    
    % Fill remaining entries with NaN
    angles = angles(1:count);
    ranges = ranges(1:count);

end

== matlab function uavPackageDelivery/On Board Computer/DataProcessing/ProcessSensorData/Visualize Point cloud ==
  data: xyzPoints input
function VisualizePointCloud(xyzPoints)
%VisualizePointCloud Display point cloud

coder.extrinsic('isOpen', 'pcplayer')

persistent player;

if isempty(player)
    % Configure axes limits
    xlimits = [-90 90];
    ylimits = [-90 90];
    zlimits = [ -50 50];
    
    % Create a streaming Lidar viewer
    player = pcplayer(xlimits, ylimits, zlimits);
end

if ~isempty(player) && isOpen(player)
    view(player, xyzPoints);
end

== matlab function uavPackageDelivery/On Board Computer/DataProcessing/ProcessSensorData/MATLAB Function ==
  data: ranges input; steerDir output; angles input; targetDir input; densityHist output
function [steerDir, densityHist] = customVFHHistogram(ranges, angles, targetDir)
%#codegen

% Enable or disable debug
debug = true;
coder.extrinsic('fprintf');
coder.extrinsic('plot_vfh_debug_plots');

% PARAMETERS
numSectors = 72;
robotRadius = 0.2;
safetyDistance = 0.1;
minTurnRadius = 0.4;
distanceLimits = [0.05 10];

%% Filter valid range readings
validIdx = (ranges > distanceLimits(1)) & (ranges < distanceLimits(2));
ranges = ranges(validIdx);
angles = angles(validIdx);

%% Create histogram
sectorEdges = linspace(-pi, pi, numSectors+1);
densityHist = zeros(1, numSectors);

for i = 1:numSectors
    inSector = (angles >= sectorEdges(i)) & (angles < sectorEdges(i+1));
    sectorRanges = ranges(inSector);

    if ~isempty(sectorRanges)
        densityHist(i) = sum(1 ./ sectorRanges);
    else
        densityHist(i) = 0;
    end
end

%% Find the steer direction
[~, targetSector] = min(abs(mod(sectorEdges(1:end-1) - targetDir + pi, 2*pi) - pi));

window = 5;
sectorRange = max(1, targetSector-window):min(numSectors, targetSector+window);

[~, minIdx] = min(densityHist(sectorRange));
steerSector = sectorRange(minIdx);

steerDir = (sectorEdges(steerSector) + sectorEdges(steerSector+1)) / 2;

%% =============================
%           DEBUGGING
% ==============================
if debug
    % Console debug (safe)
    fprintf('\n=== VFH HISTOGRAM DEBUG ===\n');
    fprintf('Valid points: %d\n', numel(ranges));
    if ~isempty(ranges)
        fprintf('Range min/max: %.2f / %.2f m\n', min(ranges), max(ranges));
    end
    fprintf('Selected sector: %d\n', steerSector);
    fprintf('Steer direction (deg): %.1f\n', steerDir * 180/pi);
    fprintf('Density (target sector): %.2f\n', densityHist(steerSector));
    fprintf('===========================\n\n');

    % % Plotting (simulation only)
    % plot_vfh_debug_plots(angles, ranges, densityHist, steerSector);
end

end
